simulink model "FSK_simulink"  (R2021a)
settings: Solver=VariableStepAuto  StartTime=0.0  StopTime=10.0  RelTol=1e-3
libraries: commdigbbndfm2 x2, dspsrcs4 x2, commchan3 x1, commsink2 x1
settings Model: Creator=kukuri  LastModifiedBy=kukuri

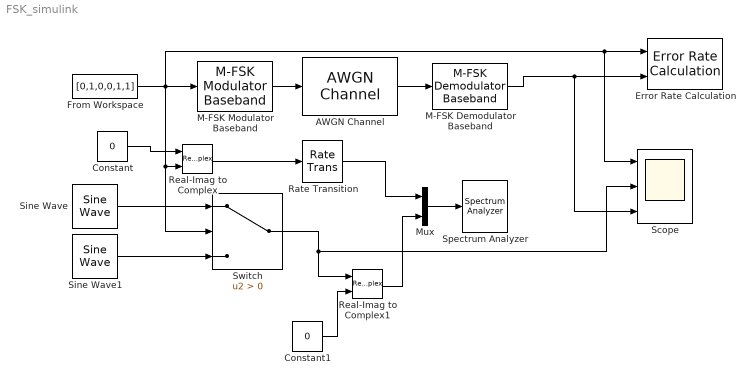
== system FSK_simulink ==
  AWGN Channel : commchan3/AWGN Channel  InputProcessing=Columns as channels (frame based)  seed=18233  noiseMode="Signal to noise ratio  (Eb/No)"  EbNodB=40  EsNodB=10  SNRdB=10  bitsPerSym=1  Ps=1  Tsym=1  variance=1
  Constant : Constant  Value=0
  Constant1 : Constant  Value=0
  Error Rate Calculation : commsink2/Error Rate Calculation  N=0  st_delay=0  cp_mode=Entire frame  subframe=[]  PMode=Workspace  WsName=ErrorVec  RsMode2=off  stop=off  numErr=100  maxBits=1e6
  From Workspace : FromWorkspace  VariableName=[0,1,0,0,1,1]  SampleTime=1/100
  M-FSK Demodulator Baseband : commdigbbndfm2/M-FSK Demodulator Baseband  M=2  OutType=Integer  Dec=Gray  freqSep=100  numSamp=40  RateOptions=Enforce single-rate processing  outDataType=double
      settings: SourceProductBaseCode=CM
  M-FSK Modulator Baseband : commdigbbndfm2/M-FSK Modulator Baseband  M=2  InType=Integer  Enc=Gray  freqSep=100  phaseType=Discontinuous  numSamp=40  RateOptions=Enforce single-rate processing  outDataType=double
  Mux : Mux  Inputs=2
  Rate Transition : RateTransition  OutPortSampleTime=1/10000
  Real-Imag to Complex : RealImagToComplex
  Real-Imag to Complex1 : RealImagToComplex
  Scope : Scope  NumInputPorts=3
  Sine Wave : dspsrcs4/Sine Wave  Amplitude=1  Frequency=3951000  Phase=0  SampleMode=Discrete  OutComplex=Real  CompMethod=Trigonometric fcn  TableSize=Speed  SampleTime=1/1000  SamplesPerFrame=1  ResetState=Restart at time zero  OutputFrames=off  dataType=double  wordLen=16  udDataType=sfix(16)  fracBitsMode=Best precision  numFracBits=15  OutDataTypeStr=double  LastOutDataTypeStr=double
  Sine Wave1 : dspsrcs4/Sine Wave  Amplitude=1  Frequency=4516000  Phase=0  SampleMode=Discrete  OutComplex=Real  CompMethod=Trigonometric fcn  TableSize=Speed  SampleTime=1/1000  SamplesPerFrame=1  ResetState=Restart at time zero  OutputFrames=off  dataType=double  wordLen=16  udDataType=sfix(16)  fracBitsMode=Best precision  numFracBits=15  OutDataTypeStr=double  LastOutDataTypeStr=double
  Spectrum Analyzer : SpectrumAnalyzer
  Switch : Switch  Criteria=u2 > Threshold
  wires:
  From Workspace/1 -> Switch/2, Real-Imag to Complex/2, Scope/1, Error Rate Calculation/1, M-FSK Modulator Baseband/1
  M-FSK Modulator Baseband/1 -> AWGN Channel/1
  AWGN Channel/1 -> M-FSK Demodulator Baseband/1
  Mux/1 -> Spectrum Analyzer/1
  Constant/1 -> Real-Imag to Complex/1
  Real-Imag to Complex/1 -> Rate Transition/1
  Rate Transition/1 -> Mux/1
  Sine Wave/1 -> Switch/1
  Sine Wave1/1 -> Switch/3
  Switch/1 -> Real-Imag to Complex1/1, Scope/2
  Constant1/1 -> Real-Imag to Complex1/2
  Real-Imag to Complex1/1 -> Mux/2
  M-FSK Demodulator Baseband/1 -> Scope/3, Error Rate Calculation/2
